simulink model "sampleModel279"  (R2021b)
settings: Solver=VariableStepAuto  StartTime=0.0  StopTime=10.0  RelTol=1e-3
undefined symbols (not defined in the file or in its folder): DiscIntNeverNeededParam
libraries: simulink x20, slpidlib x1
settings Model: Creator=user  LastModifiedBy=user

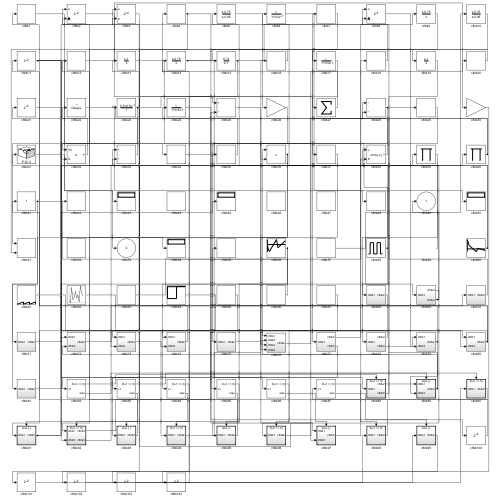
[thumbnail: Simulink's stored preview of the top-level diagram]
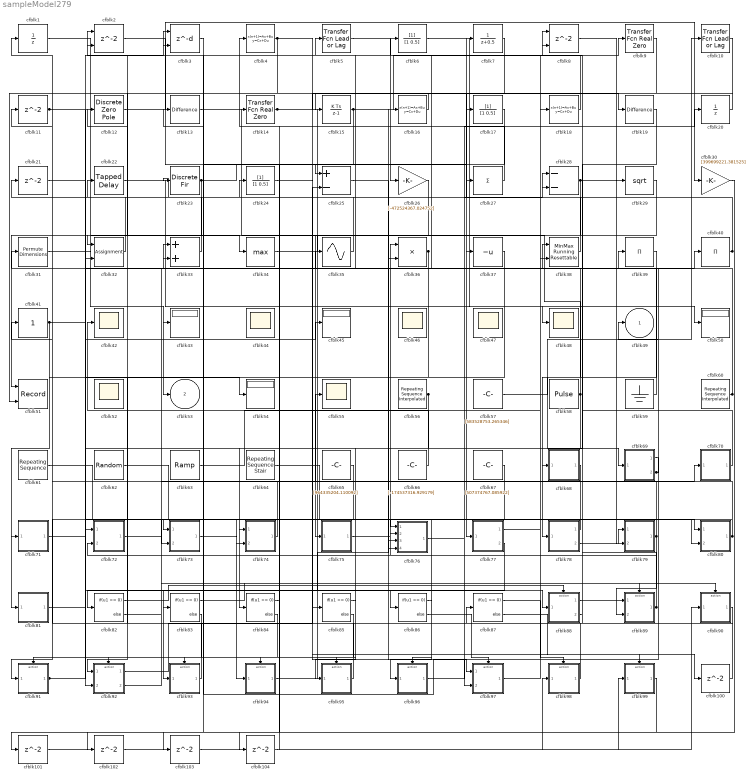
== system sampleModel279 ==
  cfblk1 : UnitDelay  HasFrameUpgradeWarning=on
  cfblk10 : simulink/Discrete/Transfer Fcn Lead or Lag  PoleZ=0.95  ZeroZ=0.75  ICPrevOutput=0.0  ICPrevInput=0.0  DoSatur=off
      settings: SourceProductBaseCode=SL
  cfblk{11,21,100..104} (7 alike) : Delay  SampleTime=1
  cfblk12 : DiscreteZeroPole  Poles=[0 0.5]  Gain=1
  cfblk13 : simulink/Discrete/Difference  ICPrevInput=0.0  OutMin=[]  OutMax=[]  OutDataTypeStr=Inherit: Inherit via back propagation  OutDataType=fixdt(1, 16)  OutScaling=2^-10  DoSatur=off
  cfblk14 : simulink/Discrete/Transfer Fcn Real Zero  ZeroZ=0.75  ICPrevInput=0.0  DoSatur=off
      settings: SourceProductBaseCode=SL
  cfblk15 : DiscreteIntegrator  ICPrevOutput=DiscIntNeverNeededParam  ICPrevScaledInput=DiscIntNeverNeededParam
  cfblk16 : DiscreteStateSpace
  cfblk17 : DiscreteFilter  SampleTime=1
  cfblk18 : DiscreteStateSpace
  cfblk19 : simulink/Discrete/Difference  ICPrevInput=0.0  OutMin=[]  OutMax=[]  OutDataTypeStr=Inherit: Inherit via back propagation  OutDataType=fixdt(1, 16)  OutScaling=2^-10  DoSatur=off
  cfblk2 : Delay  ShowEnablePort=on  SampleTime=1
      settings: InputPortMap=u0,e6
  cfblk20 : UnitDelay  HasFrameUpgradeWarning=on
  cfblk22 : simulink/Discrete/Tapped Delay  vinit=0.0  samptime=-1  NumDelays=1  DelayOrder=Oldest  includeCurrent=off
  cfblk23 : DiscreteFir  SampleTime=1
  cfblk24 : DiscreteFilter  SampleTime=1
  cfblk25 : Sum  Inputs=+-
  cfblk26 : Gain  Gain=[-472524367.024752]
  cfblk27 : Sum  Inputs=+
  cfblk28 : Sum  Inputs=--
  cfblk29 : Sqrt  SaturateOnIntegerOverflow=on
  cfblk3 : Delay  DelayLengthSource=Input port  SampleTime=1
      settings: InputPortMap=u0,p1
  cfblk30 : Gain  Gain=[399699221.381525]
  cfblk31 : PermuteDimensions
  cfblk32 : Assignment  DiagnosticForDimensions=Warning  IndexOptions=Index vector (dialog)  Indices=1  OutputSizes=1
  cfblk33 : Sum
  cfblk34 : MinMax  Function=max
  cfblk35 : Sin  TimeSource=Use external signal  SampleTime=0
  cfblk36 : Product
  cfblk37 : UnaryMinus
  cfblk38 : simulink/Math Operations/MinMax Running Resettable  Function=min  vinit=0.0
  cfblk39 : Product  Inputs=*
  cfblk4 : DiscreteStateSpace
  cfblk40 : Product  Inputs=*
  cfblk41 : simulink/Math Operations/Slider Gain  gain=1  low=0  high=2
  cfblk{42,44,46..48,52,55} (7 alike) : Scope
      cfblk44 settings: Floating=on
      cfblk46 settings: Floating=on
      cfblk47 settings: Floating=on
      cfblk52 settings: Floating=on
  cfblk{43,45,50,54} (4 alike) : Display
  cfblk5 : simulink/Discrete/Transfer Fcn Lead or Lag  PoleZ=0.95  ZeroZ=0.75  ICPrevOutput=0.0  ICPrevInput=0.0  DoSatur=off
      settings: SourceProductBaseCode=SL
  cfblk51 : Record  FileSettingsInternal="{\"entries\":[{\"content\":{\"excelSettings\":{\"content\":{},\"type\":\"Streamout.ExcelSettings\"}},\"type\":\"Streamout.FileSettingStorage\",\"uuid\":\"e13d3856-0151-4027-9874-799dcbb3d0c3\"}],\"packageUris\":[\"http://schema.mathworks.com/mf0/streamout_blocks/R2020a\"],\"version\":\"1.0\"}"  Layout=[1 1]  SignalsInternal="{\"entries\":[{\"content\":{\"signals\":[{\"content\":{\"blockPath\":[\"sampleModel279/cfblk51\"],\"channel\":[],\"dimensions\":[1],\"domain\":\"sampleModel279/cfblk51\",\"lineColor\":\"#a2142f\",\"plots\":[1],\"port\":1,\"sid\":[\"\"],\"signalID\":11815,\"signalName\":\"cfblk23\"},\"type\":\"RecordBlkView.Signal\",\"uuid\":\"6bdaff20-d8c6-4827-94f0-403183801f87\"},{\"content\":{\"blockPath\":[\"sampleModel279/cfblk51\"],\"channel\":[],\"dimensions\":[1],\"domain\":\"sampleModel279/cfblk51\",\"lineColor\":\"#139fff\",\"plots\":[1],\"port\":2,\"sid\":[\"\"],\"signalID\":11819,\"signalName\":\"cfblk7\"},\"type\":\"RecordBlkView.Signal\",\"uuid\":\"f14c097f-a958-40ef-9b6f-1fe74ddd0a89\"}]},\"type\":\"RecordBlkView.InputSignals\",\"uuid\":\"7d1fe233-e493-4734-bca6-0c7c0783f920\"}],\"packageUris\":[\"http://schema.mathworks.com/mf0/streamout_blocks/R2020a\"],\"version\":\"1.0\"}"  VisualizationBindings="{\"xyplotplugin\":{\"info\":[{\"series\":[{\"bindingParametersList\":[{\"parameter\":\"X-Axis\",\"signalID\":11815,\"signalName\":\"cfblk23\"},{\"parameter\":\"Y-Axis\",\"signalID\":11819,\"signalName\":\"cfblk7\"}],\"seriesID\":62469}],\"subplotID\":1}]}}"  CompatibilityTag=XY
  cfblk56 : simulink/Sources/Repeating Sequence Interpolated  OutValues=[-182164735.483127, -765808334.645554, 522209418.753013, -361773142.056409, 383016682.448750]  TimeValues=[0 0.1 0.5 0.6 1].'  LookUpMeth=Use Input Below  tsamp=0.01  OutMin=[]  OutMax=[]  OutDataTypeStr=double  OutputDataTypeScalingMode=double  OutDataType=fixdt(0,8)  OutScaling=2^-10
  cfblk57 : Constant  Value=[583528753.265346]  SampleTime=1
  cfblk58 : DiscretePulseGenerator  PulseType=Time based  Amplitude=[-608958195.192248]  Period=[96930117.264674]  PulseWidth=5  PhaseDelay=[9.000000]
  cfblk59 : Ground
  cfblk6 : DiscreteFilter  SampleTime=1
  cfblk60 : simulink/Sources/Repeating Sequence Interpolated  OutValues=[930794744.517939, 348475102.374012, -263397632.386348, 65145186.277425, -164664488.985096]  TimeValues=[0 0.1 0.5 0.6 1].'  LookUpMeth=Use Input Above  tsamp=0.01  OutMin=[]  OutMax=[]  OutDataTypeStr=double  OutputDataTypeScalingMode=double  OutDataType=fixdt(0,8)  OutScaling=2^-10
  cfblk61 : simulink/Sources/Repeating Sequence  rep_seq_t=[0 2]  rep_seq_y=[-501164789.220964, -445826706.779950]
  cfblk62 : UniformRandomNumber  Minimum=[-6293746588.256409]  Maximum=[2711065953.177605]  Seed=[99812368.000000]  SampleTime=0.1
  cfblk63 : simulink/Sources/Ramp  slope=[-3756.903507]  start=[37.760987]  InitialOutput=[-616633.557723]
  cfblk64 : simulink/Sources/Repeating Sequence Stair  OutValues=[-514416977.210099, 18947749.983753]  tsamp=-1  OutMin=[]  OutMax=[]  OutDataTypeStr=double  OutputDataTypeScalingMode=double  OutDataType=fixdt(0,8)  ConRadixGroup=Best Precision: Vector-wise  OutScaling=2^-12
  cfblk65 : Constant  Value=[964335204.110092]  SampleTime=1
  cfblk66 : Constant  Value=[-174537316.929179]  SampleTime=1
  cfblk67 : Constant  Value=[507374767.085922]  SampleTime=1
  cfblk68 : Subsystem
  cfblk69 : Subsystem
  cfblk7 : DiscreteTransferFcn  SampleTime=1
  cfblk70 : Subsystem
  cfblk71 : Subsystem
  cfblk72 : Subsystem
  cfblk73 : Subsystem
  cfblk74 : Subsystem
  cfblk75 : Subsystem
  cfblk76 : Subsystem
  cfblk77 : Subsystem
  cfblk78 : Subsystem
  cfblk79 : Subsystem
  cfblk8 : Delay  ShowEnablePort=on  SampleTime=1
      settings: InputPortMap=u0,e6
  cfblk80 : Subsystem
  cfblk81 : Subsystem
  cfblk{82..87} (6 alike) : If  IfExpression=u1 >= 0  SampleTime=1
  cfblk88 : Subsystem  TreatAsAtomicUnit=on
  cfblk89 : Subsystem  TreatAsAtomicUnit=on
  cfblk9 : simulink/Discrete/Transfer Fcn Real Zero  ZeroZ=0.75  ICPrevInput=0.0  DoSatur=off
      settings: SourceProductBaseCode=SL
  cfblk90 : Subsystem  TreatAsAtomicUnit=on
  cfblk91 : Subsystem  TreatAsAtomicUnit=on
  cfblk92 : Subsystem  TreatAsAtomicUnit=on
  cfblk93 : Subsystem  TreatAsAtomicUnit=on
  cfblk94 : Subsystem  TreatAsAtomicUnit=on
  cfblk95 : Subsystem  TreatAsAtomicUnit=on
  cfblk96 : Subsystem  TreatAsAtomicUnit=on
  cfblk97 : Subsystem  TreatAsAtomicUnit=on
  cfblk98 : Subsystem  TreatAsAtomicUnit=on
  cfblk99 : Subsystem  TreatAsAtomicUnit=on
  cfblk49 : Outport
  cfblk53 : Outport  Port=2
  wires:
  cfblk22/1 -> cfblk48/1
  cfblk75/1(cfblk2) -> cfblk36/1
  cfblk70/1(cfblk2) -> cfblk28/1
  cfblk41/1 -> cfblk81/1(cfblk1), cfblk33/1
  cfblk67/1 -> cfblk96/1(cfblk1)
  cfblk15/1 -> cfblk8/1, cfblk83/1
  cfblk33/1 -> cfblk23/1
  cfblk93/1(cfblk2) -> cfblk11/1
  cfblk56/1 -> cfblk84/1, cfblk95/1(cfblk1)
  cfblk13/1 -> cfblk69/1(cfblk1)
  cfblk5/1 -> cfblk26/1
  cfblk23/1 -> cfblk51/1, cfblk27/1
  cfblk77/1(cfblk2) -> cfblk18/1
  cfblk69/1(cfblk2) -> cfblk82/1
  cfblk14/1 -> cfblk86/1, cfblk19/1
  cfblk9/1 -> cfblk73/1(cfblk1)
  cfblk66/1 -> cfblk42/1
  cfblk16/1 -> cfblk15/1
  cfblk88/1(cfblk2) -> cfblk89/1(cfblk1)
  cfblk61/1 -> cfblk80/1(cfblk1)
  cfblk12/1 -> cfblk30/1
  cfblk2/1 -> cfblk25/1
  cfblk90/1(cfblk2) -> cfblk87/1
  cfblk26/1 -> cfblk75/1(cfblk1)
  cfblk77/2(cfblk5) -> cfblk93/1(cfblk1)
  cfblk10/1 -> cfblk77/1(cfblk1)
  cfblk1/1 -> cfblk34/1
  cfblk58/1 -> cfblk6/1, cfblk92/2(cfblk3)
  cfblk6/1 -> cfblk50/1
  cfblk27/1 -> cfblk4/1
  cfblk92/1(cfblk2) -> cfblk25/2
  cfblk94/1(cfblk2) -> cfblk16/1
  cfblk4/1 -> cfblk32/1, cfblk100/1
  cfblk81/1(cfblk2) -> cfblk45/1
  cfblk24/1 -> cfblk97/1(cfblk1)
  cfblk60/1 -> cfblk31/1, cfblk2/2
  cfblk62/1 -> cfblk85/1
  cfblk39/1 -> cfblk78/1(cfblk1)
  cfblk11/1 -> cfblk53/1, cfblk88/1(cfblk1), cfblk76/3(cfblk4), cfblk74/2(cfblk3)
  cfblk79/1(cfblk2) -> cfblk89/2(cfblk3), cfblk33/2
  cfblk34/1 -> cfblk37/1
  cfblk38/1 -> cfblk7/1
  cfblk89/1(cfblk2) -> cfblk38/1, cfblk76/2(cfblk3)
  cfblk35/1 -> cfblk1/1
  cfblk65/1 -> cfblk91/1(cfblk1)
  cfblk20/1 -> cfblk17/1
  cfblk73/1(cfblk2) -> cfblk94/1(cfblk1)
  cfblk96/1(cfblk2) -> cfblk20/1
  cfblk36/1 -> cfblk71/1(cfblk1), cfblk76/4(cfblk5)
  cfblk32/1 -> cfblk22/1
  cfblk72/1(cfblk2) -> cfblk70/1(cfblk1)
  cfblk37/1 -> cfblk92/1(cfblk1)
  cfblk18/1 -> cfblk2/1
  cfblk7/1 -> cfblk51/2
  cfblk21/1 -> cfblk54/1
  cfblk31/1 -> cfblk43/1
  cfblk98/1(cfblk2) -> cfblk12/1
  cfblk97/1(cfblk2) -> cfblk9/1
  cfblk78/1(cfblk2) -> cfblk76/1(cfblk1)
  cfblk95/1(cfblk2) -> cfblk13/1
  cfblk76/1(cfblk2) -> cfblk28/2
  cfblk25/1 -> cfblk97/2(cfblk5)
  cfblk63/1 -> cfblk38/2
  cfblk8/1 -> cfblk29/1
  cfblk57/1 -> cfblk10/1
  cfblk74/1(cfblk2) -> cfblk41/1
  cfblk40/1 -> cfblk24/1, cfblk3/1
  cfblk91/1(cfblk2) -> cfblk72/1(cfblk1), cfblk3/2
  cfblk59/1 -> cfblk5/1
  cfblk68/1(cfblk2) -> cfblk73/2(cfblk3)
  cfblk80/1(cfblk2) -> cfblk55/1, cfblk74/1(cfblk1), cfblk21/1
  cfblk71/1(cfblk2) -> cfblk39/1
  cfblk28/1 -> cfblk80/2(cfblk4), cfblk32/2
  cfblk92/2(cfblk4) -> cfblk40/1
  cfblk29/1 -> cfblk36/2
  cfblk78/2(cfblk4) -> cfblk79/1(cfblk1)
  cfblk88/2(cfblk5) -> cfblk72/2(cfblk3)
  cfblk19/1 -> cfblk68/1(cfblk1)
  cfblk69/2(cfblk4) -> cfblk35/1, cfblk49/1
  cfblk64/1 -> cfblk79/2(cfblk4)
  cfblk82/1 -> cfblk88/Action
  cfblk82/2 -> cfblk89/Action
  cfblk83/1 -> cfblk90/Action
  cfblk83/2 -> cfblk91/Action
  cfblk84/1 -> cfblk92/Action
  cfblk84/2 -> cfblk93/Action
  cfblk85/1 -> cfblk94/Action
  cfblk85/2 -> cfblk95/Action
  cfblk86/1 -> cfblk96/Action
  cfblk86/2 -> cfblk97/Action
  cfblk87/1 -> cfblk98/Action
  cfblk87/2 -> cfblk99/Action
  cfblk100/1 -> cfblk8/2
  cfblk30/1 -> cfblk101/1
  cfblk101/1 -> cfblk99/1(cfblk1)
  cfblk99/1(cfblk2) -> cfblk102/1
  cfblk102/1 -> cfblk98/1(cfblk1)
  cfblk3/1 -> cfblk103/1
  cfblk103/1 -> cfblk90/1(cfblk1)
  cfblk17/1 -> cfblk104/1
  cfblk104/1 -> cfblk14/1

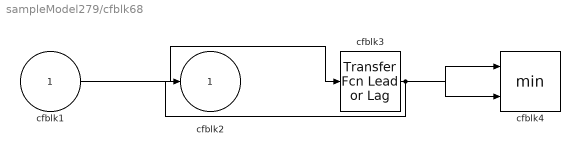
== system sampleModel279/cfblk68 ==
  cfblk1 : Inport
  cfblk3 : simulink/Discrete/Transfer Fcn Lead or Lag  PoleZ=0.95  ZeroZ=0.75  ICPrevOutput=0.0  ICPrevInput=0.0  DoSatur=off
      settings: SourceProductBaseCode=SL
  cfblk4 : MinMax  Inputs=2
  cfblk2 : Outport
  wires:
  cfblk1/1 -> cfblk3/1
  cfblk3/1 -> cfblk2/1, cfblk4/1, cfblk4/2

== system sampleModel279/cfblk69 ==
  cfblk1 : Inport
  cfblk3 : DiscreteFir  SampleTime=1
  cfblk2 : Outport
  cfblk4 : Outport  Port=2
  wires:
  cfblk1/1 -> cfblk3/1
  cfblk3/1 -> cfblk4/1, cfblk2/1

== system sampleModel279/cfblk70 ==
  cfblk1 : Inport
  cfblk3 : Bias  Bias=[-814915214.973825]
  cfblk4 : UnaryMinus
  cfblk2 : Outport
  wires:
  cfblk1/1 -> cfblk3/1
  cfblk3/1 -> cfblk4/1
  cfblk4/1 -> cfblk2/1

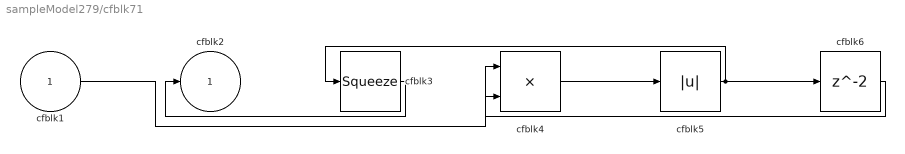
== system sampleModel279/cfblk71 ==
  cfblk1 : Inport
  cfblk3 : Squeeze
  cfblk4 : Product
  cfblk5 : Abs
  cfblk6 : Delay  SampleTime=1
  cfblk2 : Outport
  wires:
  cfblk4/1 -> cfblk5/1
  cfblk5/1 -> cfblk3/1, cfblk6/1
  cfblk3/1 -> cfblk2/1
  cfblk1/1 -> cfblk4/1
  cfblk6/1 -> cfblk4/2

== system sampleModel279/cfblk72 ==
  cfblk1 : Inport
  cfblk3 : Inport  Port=2
  cfblk2 : Outport
  wires:
  cfblk1/1 -> cfblk2/1

== system sampleModel279/cfblk73 ==
  cfblk1 : Inport
  cfblk3 : Inport  Port=2
  cfblk2 : Outport
  wires:
  cfblk3/1 -> cfblk2/1

== system sampleModel279/cfblk74 ==
  cfblk1 : Inport
  cfblk3 : Inport  Port=2
  cfblk2 : Outport
  wires:
  cfblk3/1 -> cfblk2/1

== system sampleModel279/cfblk75 ==
  cfblk1 : Inport
  cfblk3 : simulink/Discrete/Transfer Fcn First Order  PoleZ=0.95  ICPrevOutput=0.0  DoSatur=off
  cfblk2 : Outport
  wires:
  cfblk1/1 -> cfblk3/1
  cfblk3/1 -> cfblk2/1

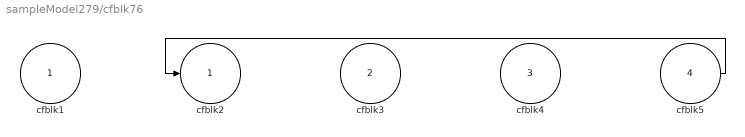
== system sampleModel279/cfblk76 ==
  cfblk1 : Inport
  cfblk3 : Inport  Port=2
  cfblk4 : Inport  Port=3
  cfblk5 : Inport  Port=4
  cfblk2 : Outport
  wires:
  cfblk5/1 -> cfblk2/1

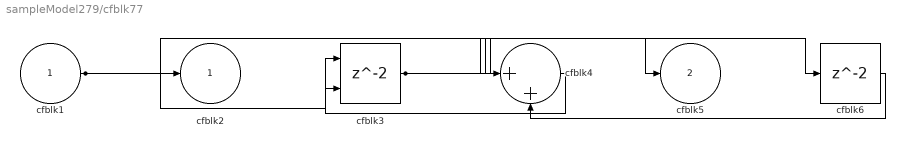
== system sampleModel279/cfblk77 ==
  cfblk1 : Inport
  cfblk3 : Delay  ShowEnablePort=on  SampleTime=1
      settings: InputPortMap=u0,e6
  cfblk4 : Sum  Inputs=|++
  cfblk6 : Delay  SampleTime=1
  cfblk2 : Outport
  cfblk5 : Outport  Port=2
  wires:
  cfblk3/1 -> cfblk5/1, cfblk6/1
  cfblk1/1 -> cfblk2/1, cfblk4/1, cfblk3/2
  cfblk4/1 -> cfblk3/1
  cfblk6/1 -> cfblk4/2

== system sampleModel279/cfblk78 ==
  cfblk1 : Inport
  cfblk3 : Constant  Value=[-950045351.686305]  SampleTime=1
  cfblk2 : Outport
  cfblk4 : Outport  Port=2
  wires:
  cfblk3/1 -> cfblk2/1
  cfblk1/1 -> cfblk4/1

== system sampleModel279/cfblk79 ==
  cfblk1 : Inport
  cfblk4 : Inport  Port=2
  cfblk3 : Sum  Inputs=+
  cfblk2 : Outport
  wires:
  cfblk4/1 -> cfblk2/1
  cfblk1/1 -> cfblk3/1

== system sampleModel279/cfblk80 ==
  cfblk1 : Inport
  cfblk4 : Inport  Port=2
  cfblk3 : Sum  Inputs=+-
  cfblk2 : Outport
  wires:
  cfblk1/1 -> cfblk3/1, cfblk3/2
  cfblk4/1 -> cfblk2/1

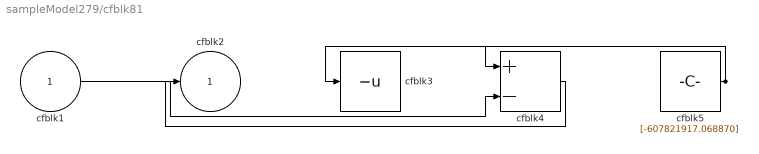
== system sampleModel279/cfblk81 ==
  cfblk1 : Inport
  cfblk3 : UnaryMinus
  cfblk4 : Sum  Inputs=+-
  cfblk5 : Constant  Value=[-607821917.068870]  SampleTime=1
  cfblk2 : Outport
  wires:
  cfblk5/1 -> cfblk4/1, cfblk3/1
  cfblk1/1 -> cfblk4/2
  cfblk4/1 -> cfblk2/1

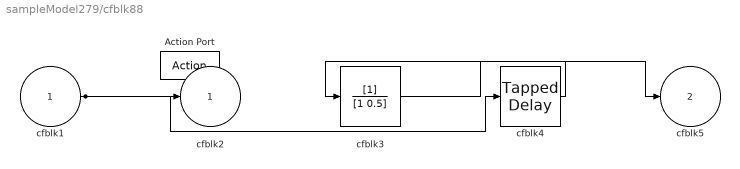
== system sampleModel279/cfblk88 ==
  cfblk1 : Inport
  Action Port : ActionPort  ActionPortLabel=if(u1 >= 0)
  cfblk3 : DiscreteFilter
  cfblk4 : simulink/Discrete/Tapped Delay  vinit=0.0  samptime=-1  NumDelays=1  DelayOrder=Oldest  includeCurrent=off
  cfblk2 : Outport
  cfblk5 : Outport  Port=2
  wires:
  cfblk4/1 -> cfblk3/1
  cfblk1/1 -> cfblk4/1, cfblk2/1
  cfblk3/1 -> cfblk5/1

== system sampleModel279/cfblk89 ==
  cfblk1 : Inport
  cfblk3 : Inport  Port=2
  Action Port : ActionPort  ActionPortLabel=else
  cfblk2 : Outport
  wires:
  cfblk3/1 -> cfblk2/1

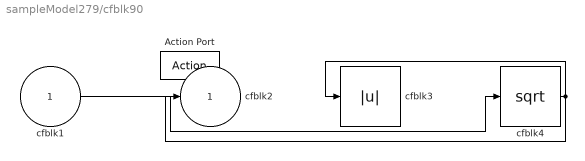
== system sampleModel279/cfblk90 ==
  cfblk1 : Inport
  Action Port : ActionPort  ActionPortLabel=if(u1 >= 0)
  cfblk3 : Abs
  cfblk4 : Sqrt  SaturateOnIntegerOverflow=on
  cfblk2 : Outport
  wires:
  cfblk1/1 -> cfblk4/1
  cfblk4/1 -> cfblk2/1, cfblk3/1

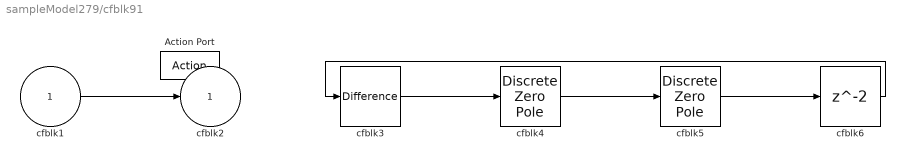
== system sampleModel279/cfblk91 ==
  cfblk1 : Inport
  Action Port : ActionPort  ActionPortLabel=else
  cfblk3 : simulink/Discrete/Difference  ICPrevInput=0.0  OutMin=[]  OutMax=[]  OutDataTypeStr=Inherit: Inherit via back propagation  OutDataType=fixdt(1, 16)  OutScaling=2^-10  DoSatur=off
  cfblk4 : DiscreteZeroPole  Poles=[0 0.5]  Gain=1  SampleTime=-1
  cfblk5 : DiscreteZeroPole  Poles=[0 0.5]  Gain=1  SampleTime=-1
  cfblk6 : Delay
  cfblk2 : Outport
  wires:
  cfblk1/1 -> cfblk2/1
  cfblk4/1 -> cfblk5/1
  cfblk3/1 -> cfblk4/1
  cfblk5/1 -> cfblk6/1
  cfblk6/1 -> cfblk3/1

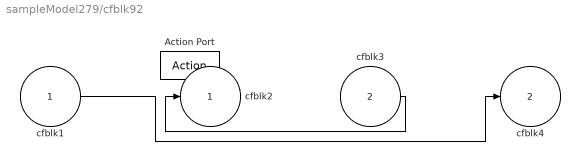
== system sampleModel279/cfblk92 ==
  cfblk1 : Inport
  cfblk3 : Inport  Port=2
  Action Port : ActionPort  ActionPortLabel=if(u1 >= 0)
  cfblk2 : Outport
  cfblk4 : Outport  Port=2
  wires:
  cfblk3/1 -> cfblk2/1
  cfblk1/1 -> cfblk4/1

== system sampleModel279/cfblk93 ==
  cfblk1 : Inport
  Action Port : ActionPort  ActionPortLabel=else
  cfblk3 : Sqrt  SaturateOnIntegerOverflow=on
  cfblk2 : Outport
  wires:
  cfblk1/1 -> cfblk2/1, cfblk3/1

== system sampleModel279/cfblk94 ==
  cfblk1 : Inport
  Action Port : ActionPort  ActionPortLabel=if(u1 >= 0)
  cfblk3 : Constant  Value=[943492305.523102]  SampleTime=1
  cfblk2 : Outport
  wires:
  cfblk3/1 -> cfblk2/1

== system sampleModel279/cfblk95 ==
  cfblk1 : Inport
  Action Port : ActionPort  ActionPortLabel=else
  cfblk3 : simulink/Discrete/Transfer Fcn Real Zero  ZeroZ=0.75  ICPrevInput=0.0  DoSatur=off
      settings: SourceProductBaseCode=SL
  cfblk2 : Outport
  wires:
  cfblk1/1 -> cfblk3/1
  cfblk3/1 -> cfblk2/1

== system sampleModel279/cfblk96 ==
  cfblk1 : Inport
  Action Port : ActionPort  ActionPortLabel=if(u1 >= 0)
  cfblk3 : slpidlib/PID Controller  Controller=PID  Form=Parallel  TimeDomain=Discrete-time  UseExternalTs=off  SampleTime=-1  IntegratorMethod=Forward Euler  FilterMethod=Forward Euler  ControllerParametersSource=internal  P=1  I=1  D=0  UseFilter=on  N=100  TunerSelectOption=Transfer Function Based (PID Tuner App)  InitialConditionSource=internal  InitialConditionForIntegrator=0  InitialConditionForFilter=0  DifferentiatorICPrevScaledInput=0  ExternalReset=none  TrackingMode=off  Kt=1  LimitOutput=off  SatLimitsSource=internal  UpperSaturationLimit=inf  LowerSaturationLimit=-inf  LinearizeAsGain=off  AntiWindupMode=none  Kb=1  POutMin=[]  POutMax=[]  IOutMin=[]  IOutMax=[]  DOutMin=[]  DOutMax=[]  NOutMin=[]  NOutMax=[]  SumOutMin=[]  SumOutMax=[]  SaturationOutMin=[]  SaturationOutMax=[]  PParamMin=[]  PParamMax=[]  IParamMin=[]  IParamMax=[]  DParamMin=[]  DParamMax=[]  NParamMin=[]  NParamMax=[]  KbParamMin=[]  KbParamMax=[]  KtParamMin=[]  KtParamMax=[]  KbOutMin=[]  KbOutMax=[]  KtOutMin=[]  KtOutMax=[]  IntegratorOutMin=[]  IntegratorOutMax=[]  FilterOutMin=[]  FilterOutMax=[]  SumI1OutMin=[]  SumI1OutMax=[]  SumI2OutMin=[]  SumI2OutMax=[]  SumI3OutMin=[]  SumI3OutMax=[]  SumI4OutMin=[]  SumI4OutMax=[]  SumDOutMin=[]  SumDOutMax=[]  DifferentiatorOutMin=[]  DifferentiatorOutMax=[]  FilterDiffOutCoefMin=[]  FilterDiffOutCoefMax=[]  ReciprocalOutMin=[]  ReciprocalOutMax=[]  SumDenOutMin=[]  SumDenOutMax=[]  SumNumOutMin=[]  SumNumOutMax=[]  DivideOutMin=[]  DivideOutMax=[]  UdiffTsProdOutMin=[]  UdiffTsProdOutMax=[]  NTsProdOutMin=[]  NTsProdOutMax=[]  UintegralTsProdOutMin=[]  UintegralTsProdOutMax=[]  UngainTsProdOutMin=[]  UngainTsProdOutMax=[]  IntegratorContinuousStateAttributes=''  IntegratorStateMustResolveToSignalObject=off  IntegratorRTWStateStorageClass=Auto  FilterContinuousStateAttributes=''  FilterStateMustResolveToSignalObject=off  FilterRTWStateStorageClass=Auto  ParallelPVariant=InternalParameters  IdealPVariant=Disabled  IVariant=InternalParameters  DVariant=InternalParameters  IntegratorVariant=Discrete  SatVariant=Disabled  AWVariant=Passthrough  PCopyVariant=Disabled  TRVariant=Disabled  FdbkBlocksVariant=Forward  IdealPFdbkVariant=Disabled  SatFdbkVariant=Disabled  DerivativeFilterVariant=ForwardEulerFilter  NVariant=InternalParameters  NCopyVariant=Disabled  FilterICVariant=InternalICsFilter  IntegratorICVariant=InternalICs  ExternalResetVariant=Disabled  TRSumVariant=Passthrough  SumFdbkVariant=Disabled  SumVariant=Sum_PID  TsampFilterVariant=InternalTs  TsampNgainVariant=Passthrough  TsampIntegralVariant=Passthrough  ExternalSaturationOutDataTypeStr=Inherit: Same as second input
  cfblk2 : Outport
  wires:
  cfblk1/1 -> cfblk3/1
  cfblk3/1 -> cfblk2/1

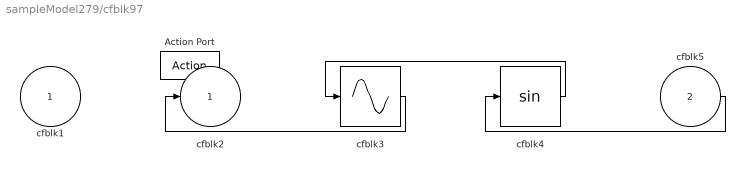
== system sampleModel279/cfblk97 ==
  cfblk1 : Inport
  cfblk5 : Inport  Port=2
  Action Port : ActionPort  ActionPortLabel=else
  cfblk3 : Sin  TimeSource=Use external signal  SampleTime=0
  cfblk4 : Trigonometry
  cfblk2 : Outport
  wires:
  cfblk3/1 -> cfblk2/1
  cfblk4/1 -> cfblk3/1
  cfblk5/1 -> cfblk4/1

== system sampleModel279/cfblk98 ==
  cfblk1 : Inport
  Action Port : ActionPort  ActionPortLabel=if(u1 >= 0)
  cfblk3 : DiscreteFilter
  cfblk2 : Outport
  wires:
  cfblk1/1 -> cfblk3/1
  cfblk3/1 -> cfblk2/1

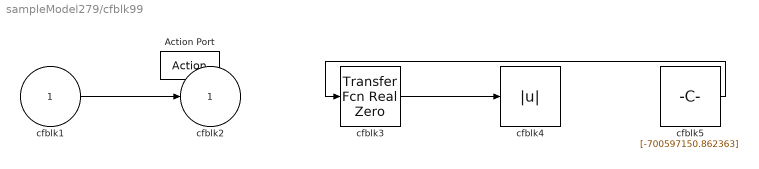
== system sampleModel279/cfblk99 ==
  cfblk1 : Inport
  Action Port : ActionPort  ActionPortLabel=else
  cfblk3 : simulink/Discrete/Transfer Fcn Real Zero  ZeroZ=0.75  ICPrevInput=0.0  DoSatur=off
      settings: SourceProductBaseCode=SL
  cfblk4 : Abs
  cfblk5 : Constant  Value=[-700597150.862363]  SampleTime=1
  cfblk2 : Outport
  wires:
  cfblk5/1 -> cfblk3/1
  cfblk1/1 -> cfblk2/1
  cfblk3/1 -> cfblk4/1
